simulink model "Prescan_Carsim_0118_repair_cs"  (R2019b)
settings: Solver=ode5  StartTime=0.0  StopTime=inf  FixedStep=1/1000  RelTol=1e-3
PreLoadFcn:
  | mbxruntime.callbacks.PreLoadFcn(bdroot);
PostLoadFcn:
  | mbxruntime.callbacks.PostLoadFcn(bdroot);
InitFcn:
  | mbxruntime.callbacks.InitFcn(bdroot);
  | Initialization_Func;
  | %T01_Init_2106;
StartFcn:
  | mbxruntime.callbacks.StartFcn(bdroot);
  | current_sys=gcs;
  | speedblock=Simulink.findBlocks(current_sys,'Name','speed_kmh_Gain');
  | h1=add_exec_event_listener(speedblock,'PostOutputs',@SpeedVisulization);
  | outblock=Simulink.findBlocks(current_sys,'Name','trajectorycurveoutput_Gain');
  | CurveTrajectoryListenerHandle=add_exec_event_listener(outblock,'PostOutputs',@TrajectoryCurve_CallBack);
  | lanedatablock=Simulink.findBlocks(current_sys,'Name','LaneData_Gain');
  | CurveLaneListenerHandle=add_exec_event_listener(lanedatablock,'PostOutputs',@CurveLane_CallBack);
StopFcn:
  | mbxruntime.callbacks.StopFcn(bdroot);
model workspace: external: MAT-File .\Prescan_Carsim_1230_cs_hws.mat (data not in the file)
undefined symbols (not defined in the file or in its folder): AAx, AAy, AAz, AVx, AVy, AVz, Ax, Ay, Az, canChannel, DiscIntNeverNeededParam, g, InitialDPMPDF_Comfort, InitialDPMPDF_Efficiency, InitialDPMPDF_Safety, InitialPDF_DEM, InitialPlanningParameter, Kf, Kr, Lr, M, mbxruntime, nG, NormalisedTrajectoryIndicator_Pool, Parameter_Indicator_LookUpTable, Prescan_Carsim_1230_cs_0658e9ca1334a8be, Prescan_Carsim_1230_cs_08c5eb9a1bd7376a, Prescan_Carsim_1230_cs_6cfd759b89b9fc85, Prescan_Carsim_1230_cs_9435cc1cceb5050d, Prescan_Carsim_1230_cs_ac716d34d49f74ab, Prescan_Carsim_1230_cs_be02757d7f212dd5, Rational_Coefficient_Learning, SteeringWheel, TrajectoryIndicatorRange, V, VehicleBaseLength, Vx, Vy, Vz, WheelL0, WheelL1, WheelR0, WheelR1
libraries: canmsglib x11, dsparch4 x6, canlib x3, PreScanSimulinkLibrary x3, Solver_SF x1, autolibshared x1
(part 5 of 8)

== matlab function Prescan_Carsim_0118_repair_cs/BMW_X5_SUV_1/trajectory planning/Road data extraction ==
  data: RoadLanePoly_Rotation output; RoadLaneEnd_Rotation output; u input; PathLength_Planning input; RoadLane_Plan output double size=[1000 4]; Interval_RoadSegment input; Width_Road input
function [RoadLanePoly_Rotation,RoadLaneEnd_Rotation,RoadLane_Plan]=fcn(u,PathLength_Planning,Interval_RoadSegment,Width_Road)
% calculate the road based on the ALMS sensor
% #codegen

Labels=zeros(size(u,1) , 1);
Lengths = zeros(size(u,1) , 1);
GroupIDs = zeros(size(u,1) , 1);
Pxs = zeros(size(u,1) , 4);
Pys = zeros(size(u,1) , 4);

for i = 1 : size(u,1)  
    % The valid parameter indicates that the data slot in the bus is actually filled in
    if u(i).HEADER.valid == 1         
        Labels(i)=u(i).DATA.LineLabel;
        Lengths(i) = u(i).DATA.Length; 
        GroupIDs(i) =u(i).DATA.GroupID;       
        % Count the number of groups. Polynomials with the same GroupID are
        % published sequentially in the output, which allows us to use this
        % simple piece of code.       
        % Construct polynomial definitions 
        Pxs(i,:) = [u(i).DATA.X.N3, u(i).DATA.X.N2, u(i).DATA.X.N1, u(i).DATA.X.N0];
        Pys(i,:) = [u(i).DATA.Y.N3, u(i).DATA.Y.N2, u(i).DATA.Y.N1, u(i).DATA.Y.N0];        
    end  
end

%Left Lane
ID_Left_Lane=find(Labels==5);% the left lane is labels as 5
%Right Lane
ID_Right_Lane=find(Labels==4);% the right lane is labels as 4

% Align the left and right raod lane and cut into segments with fixed
% intervals.

% To use the path planning method, we need to Align  of Left and Right Lane.
% Method 1: Cut by the Cross Dot method by Aligning the Road_Start & the
% Road_End

% Method 2:Make a Virtual Lane with a fixed Road Width 3.75m and a fixed 
% Lane Length(==PathLength_Planning)to the Base Line.
%{
% S1,Estimate the Direction of the foward Road and to determine the Base Lane
% Direction Estimation Method:the Whole Lane is on the one side of the
% vehicle longitudinal axis 
% if Flag_Left==1, the Whole Left Lane is on the left of the vehicle
Vec_Left_Lane=[LeftLane_Vis,zeros(Num_Left,1)];
Cross_LongidVehicleAxisToLeftLane=cross(Vec_LongidVehicleAxis,Vec_Left_Lane);
Flag_Left=all(Cross_LongidVehicleAxisToLeftLane(:,3)>0);

% if Flag_Right==1, the Whole Right Lane is on the right of the vehicle
Vec_Right_Lane=[RightLane_Vis,zeros(Num_Left,1)];
Cross_LongidVehicleAxisToLeftLane=cross(Vec_LongidVehicleAxis,Vec_Right_Lane);
Flag_Right=all(Cross_LongidVehicleAxisToLeftLane(:,3)<0);
% Notice that: the Lane data coordinates is the Vehicle Coordination.
%}

% Step 1,If RightLane longer than the Path_length_Planning,Choose the Right 
% one,otherwise,choose the longer one. 
% Step 2, made the Virtual Lane with a fixed Road Width 3.75m
% LeftLane_Plan=zeros(1000,2);
% RightLane_Plan=zeros(1000,2);
Length_RightLane=sum(Lengths(ID_Right_Lane));
Length_LeftLane=sum(Lengths(ID_Left_Lane));
if Length_RightLane<PathLength_Planning && Length_RightLane<Length_LeftLane
    Flag_RightBase=0;
    if Length_LeftLane>PathLength_Planning
        %LeftLane is longer than PathLength_Planning
        [LeftLane_PlanTemp,Num_LeftLane]=RoadLane_Extract_Plan(ID_Left_Lane,Pxs,Pys,Lengths,PathLength_Planning,Interval_RoadSegment);    
    else
        [LeftLane_PlanTemp,Num_LeftLane]=RoadLane_Extract_Plan(ID_Left_Lane,Pxs,Pys,Lengths,Length_LeftLane,Interval_RoadSegment);
    end
    LeftLane_Plan=LeftLane_PlanTemp(1:Num_LeftLane,:);
    [RightLane_Plan]=Made_VirtualLane(LeftLane_Plan,Flag_RightBase,Width_Road);
else
    Flag_RightBase=1;
    if Length_RightLane>PathLength_Planning
        [RightLane_PlanTemp,Num_RightLane]=RoadLane_Extract_Plan(ID_Right_Lane,Pxs,Pys,Lengths,PathLength_Planning,Interval_RoadSegment);     
    else
        [RightLane_PlanTemp,Num_RightLane]=RoadLane_Extract_Plan(ID_Right_Lane,Pxs,Pys,Lengths,Length_RightLane,Interval_RoadSegment);
    end
    RightLane_Plan=RightLane_PlanTemp(1:Num_RightLane,:);
    [LeftLane_Plan]=Made_VirtualLane(RightLane_Plan,Flag_RightBase,Width_Road);
end

RoadLane_Plan=[LeftLane_Plan,RightLane_Plan];

% Fit the RoadLane 
Order_polyfit=6;
rotationangle=deg2rad(45);
rotationmatrix=[cos(rotationangle),sin(rotationangle);-sin(rotationangle),cos(rotationangle)];
leftlane_rotation=LeftLane_Plan*rotationmatrix;
Poly_LeftRotation=polyfit(leftlane_rotation(:,1),leftlane_rotation(:,2),Order_polyfit);
rightlane_rotation=RightLane_Plan*rotationmatrix;
Poly_RightRotation=polyfit(rightlane_rotation(:,1),rightlane_rotation(:,2),Order_polyfit);
RoadLanePoly_Rotation=[Poly_LeftRotation',Poly_RightRotation'];
RoadLaneEnd_Rotation=[leftlane_rotation(end,:),rightlane_rotation(end,:)];

end

%%
% Local functions
function [Temp_Lane,Num_Lane]=RoadLane_Extract_Vis(ID_Lane,Num_short_length,Pxs,Pys,Lengths)
% Extract Lane data according to the Polyvals from ALMS
% Input: 
%   Num_short_length, when the road length of a poly short than this 
%       this value, the polyval is evaluated with a smaller interval
%   Pxs,Pys, the poly coefficients for X,Y
Temp_Lane=zeros(5000,2);% a large vector used to store the data
Num_Lane=0;
for i=1:length(ID_Lane)
    road_length=Lengths(ID_Lane(i)); 
    if road_length<1
        L = linspace(0,road_length,Num_short_length);
    else
        L = 0:0.1:road_length;
    end        
    X_temp = polyval(Pxs(ID_Lane(i),:),L);
    Y_temp = polyval(Pys(ID_Lane(i),:),L);        
    Num_point=length(L);        
    Temp_Lane(Num_Lane+1:Num_Lane+Num_point,1)=X_temp';
    Temp_Lane(Num_Lane+1:Num_Lane+Num_point,2)=Y_temp';
    Num_Lane=Num_Lane+Num_point;
end
end

function [Lane_Plan,Num_RoadSegment]=RoadLane_Extract_Plan(ID_Lane,Pxs,Pys,Lengths,LaneLength,Interval_RoadSegment)
% Extract Lane data according to the Polyvals from ALMS
% Input: 
%   Pxs,Pys, the poly coefficients for X,Y
%   PathLength, the target path length 
%   Interval_RoadSegmetn,choose the raod point with a length interval.
Lane_Plan=zeros(1000,2);
LengthPoint=0:Interval_RoadSegment:LaneLength;
Num_RoadSegment=length(LengthPoint);
CumSum_LengthLane=cumsum([0;Lengths(ID_Lane)]);
% the First Road segment point
Lane_Plan(1,1)= polyval(Pxs(ID_Lane(1),:),0);
Lane_Plan(1,2)= polyval(Pys(ID_Lane(1),:),0); 
for i=2:Num_RoadSegment
    LengthPoint_i=LengthPoint(i);
    ID_Close=find(LengthPoint_i<=CumSum_LengthLane);
    ID_poly=ID_Close(1,1)-1;        
    Lane_Plan(i,1) = polyval(Pxs(ID_Lane(ID_poly),:),LengthPoint_i-CumSum_LengthLane(ID_poly));
    Lane_Plan(i,2) = polyval(Pys(ID_Lane(ID_poly),:),LengthPoint_i-CumSum_LengthLane(ID_poly));                       
end
end

function [Lane_Virtual]=Made_VirtualLane(BaseLane,Flag_RightBase,Width_Road)
% made the virtual lane based on the baselane with a fixed road width
% 3.75m.
% BaseLane: a array like Num_roadpoint*2,the first column is the X
% coordinates while the other column is the Y coordinates.
% Flag_Right:a logical variable, if 1, it shows the baselane is the right
% one, if 0, the baselane is the left one.
% Lane_Virtual=zeros(1000,2);% a large data array to fix the size of the output.
Vec_BaseLane=zeros(size(BaseLane,1),2);
Vec_BaseLane(1:end-1,1)=BaseLane(2:end,1)-BaseLane(1:end-1,1);
Vec_BaseLane(end,1)=Vec_BaseLane(end-1,1);
Vec_BaseLane(1:end-1,2)=BaseLane(2:end,2)-BaseLane(1:end-1,2);
Vec_BaseLane(end,2)=Vec_BaseLane(end-1,2);
VecLength_BaseLane=sqrt(Vec_BaseLane(:,1).^2+Vec_BaseLane(:,2).^2);
Vec_BaseLane_unit=[Vec_BaseLane(:,1)./VecLength_BaseLane,Vec_BaseLane(:,2)./VecLength_BaseLane];
if Flag_RightBase==1
    Rotation_Transformation=[0,-1;1,0];
else
    Rotation_Transformation=[0,1;-1,0];
end
Vec_VirtualToBase=Rotation_Transformation*Vec_BaseLane_unit';% 2*N
Lane_Virtual=BaseLane+Width_Road*Vec_VirtualToBase';

end



%{
function [Flag_Cut,SecondLane_AfterCut]=Road_Align(FirstLane,SecondLane,Rotation_Angle_deg)
% Function:Align the Road_Start & the Road_End
% Method: Cut by the Cross Dot method
% Input: Rotation_Angle=90 for the FirstLane is the Right lane;
%        Rotation_Angle=-90 for the FirstLane is the Left lane.
%        FisrtLane or SecondLane is a data array like Num*2, the first column is the X
%        coordinates,and the second column is the Y coordinates.
Num_Second=size(SecondLane,1);

Vec_First_Start=zeros(1,3);
Vec_First_Start(1,1:2)=FirstLane(2,:)-FirstLane(1,:);
% clock-wise (Negative) for Left Lane to rotate
% Rotation_Angle=deg2rad(-90);
% Rotation_Angle=deg2rad(Rotation_Angle_deg);
Rotation_Transformation=[cos(Rotation_Angle),-1*sin(Rotation_Angle);sin(Rotation_Angle),cos(Rotation_Angle)];

Vec_SecondToFirstStart=zeros(Num_Second,3);
Vec_SecondToFirstStart(:,1:2)=SecondLane-FirstLane(1,:);

Vec_VerticalToFirstStart=[Rotation_Transformation*Vec_First_Start(1,1:2)';0];
Vec_VerticalToFirstStart_Matrix=repmat(Vec_VerticalToFirstStart',Num_Second,1);
Cross_VerticalToLeftStart=cross(Vec_VerticalToFirstStart_Matrix,Vec_SecondToFirstStart);
% Find the road point that lies out of the Vec_VerticalToLeftStart
ID_FirstStart=find(Cross_VerticalToLeftStart(:,3)*sign(Rotation_Angle)>0);
if isempty(ID_FirstStart)
    Flag_Cut=0;    
    SecondLane_AfterCut=SecondLane;
else
    Flag_Cut=1;
    SecondLane_AfterCut=SecondLane(ID_FirstStart(end)+1:end,:);   
end
end
%}

== matlab function Prescan_Carsim_0118_repair_cs/BMW_X5_SUV_1/Tracking Control & vehicle dynamics/Lane Keeping Assistance/Path Tracking - LQR controller/LQR Feedforward ==
  data: Feedforward output; PreviewDistance input; Curvature input; v input
function Feedforward = fcn(PreviewDistance, Curvature,v)
% LQR前馈量计算，与赵斌的SMC前馈量计算完全一致
%先定义车辆本身的参数
g=9.8;%重力加速度m/s^2

%=============== Original Vehicle Parameters
M=1396; %车辆的质量kg
I=2204; %车辆的横摆转动惯量kg·m2
Kf=50192; %前轮的侧偏刚度Nm/rad
Kr=50192; %后轮的侧偏刚度Nm/rad
Lf=1.01; %车辆质心到前轴的距离m
Lr=1.59; %车辆质心到后轴的距离m
%{
%=====The JTEKT vehicle Parameter
M=1275; %车辆的质量kg
I=1523; %车辆的横摆转动惯量kg·m2
Kf=20000; %Calculated According to the carsim vehicle tire (under Fn=3500N)
Kr=20000; %后轮的侧偏刚度Nm/rad
Lf=1.016; %车辆质心到前轴的距离m
Lr=1.644; %车辆质心到后轴的距离m
%}


%待调参数： 预瞄时长t_pre, 滑膜面参数 c1, c2, 趋近率参数delta, kapa
%输入参数； 预瞄偏差ep,  参考航向角phi_d, 本车航向角 phi, 道路曲率 qulv  航向角偏差影响系数 phir_k0 phir_k1
L = PreviewDistance; %车辆预瞄距离设定
smc_a34 = (Kf+Kr)/M+L*(Kf*Lf-Kr*Lr)/I;
smc_b32 = (L*Kf*Lf)/I+Kf/M;
k3 = smc_a34/smc_b32;
Feedforward= (M*v^2*Curvature)/(2*(Lf+Lr))*(Lr/Kf-Lf/Kr+Lf/Kr*k3)+Curvature*((Lf+Lr)-Lr*k3);

== matlab function Prescan_Carsim_0118_repair_cs/BMW_X5_SUV_1/trajectory planning/Specific Curve Trajectory Planning/Trajectory Planning For Curve under beginning-global/Trajectory Planning For Curve ==
  data: RoadLane_Plan input size=[1000 4]; PathPlan_Global output size=[1000 2]; Parameter_TrajectoryPlan input size=[9 1]; Speed_Planned_kmh output size=[1000 1]; VehicleWidth input; LaneWidth input; PlanPathDataLength_Curve output size=1; VehicleState_Beginning input
function [PathPlan_Global,Speed_Planned_kmh,PlanPathDataLength_Curve]= fcn(RoadLane_Plan,Parameter_TrajectoryPlan,VehicleWidth,LaneWidth,VehicleState_Beginning)
%Road Lane
Path_PlanTemp=zeros(1000,2);
Num_LanePlan=size(RoadLane_Plan,1);
LeftLane_Plan=RoadLane_Plan(:,1:2);
RightLane_Plan=RoadLane_Plan(:,3:4);
X_LaneLeftToRight=RightLane_Plan(:,1)-LeftLane_Plan(:,1);
Y_LaneLeftToRight=RightLane_Plan(:,2)-LeftLane_Plan(:,2);
Vec_LeftToRight=[X_LaneLeftToRight,Y_LaneLeftToRight];
LaneWidth_Estimated=sqrt(sum(Vec_LeftToRight.*Vec_LeftToRight,2));
UnitVec_LeftRight=Vec_LeftToRight./[LaneWidth_Estimated,LaneWidth_Estimated];
LaneCenter=zeros(Num_LanePlan,2);
LaneCenter(:,1)=0.5*(LeftLane_Plan(:,1)+RightLane_Plan(:,1));
LaneCenter(:,2)=0.5*(LeftLane_Plan(:,2)+RightLane_Plan(:,2));
LeftBound=LaneCenter-(LaneWidth-VehicleWidth)*0.5*UnitVec_LeftRight; % The Path Bound Should consider the Vehicle Width
RightBound=LaneCenter+(LaneWidth-VehicleWidth)*0.5*UnitVec_LeftRight;

%path planning
% Trajectory planning parameters
Init_pos=0.5;
Parameter_PathPlan=Parameter_TrajectoryPlan(1:4,1);
if sum(Parameter_TrajectoryPlan(1:3)>1)
    Parameter_PathPlan=[0,0,1,0.5];
end
% if Parameter_PathPlan(3)==1
%     alpha=ones(Num_LanePlan,1)*Parameter_PathPlan(4);
%     alpha(1:2)=Init_pos;
%     alpha(end-1:end)=Init_pos;  
% else
[alpha_path_length,alpha_curvature,~,~,G]= PathPlanning(RightBound(:,1),...
    RightBound(:,2),LeftBound(:,1),LeftBound(:,2),Init_pos);
% fixed lateral offst
alpha_fixlatoff=ones(Num_LanePlan,1)*Parameter_PathPlan(4);
sign_center=sign(Parameter_PathPlan(4)-Init_pos);
offset=0.02;
alpha_fixlatoff(1:3)=Init_pos;% consistent within the pathplanning function
alpha_fixlatoff(4:21)=pchip([1,5,14,18],[Init_pos,Init_pos+sign_center*offset,Parameter_PathPlan(4)-sign_center*offset,Parameter_PathPlan(4)],(1:18));
alpha_fixlatoff(end-2:end)=Init_pos;
% alpha_heading(4:6)=spline([1,5],[Init_pos,Parameter_PathPlan(4)],(2:4));
% alpha_heading(end-5:end-3)=spline([1,5],[Parameter_PathPlan(4),Init_pos],(2:4));
alpha_fixlatoff(end-20:end-3)=pchip([1,5,14,18],[Parameter_PathPlan(4),Parameter_PathPlan(4)-sign_center*offset,Init_pos+sign_center*offset,Init_pos],(1:18));

alpha=[alpha_path_length,alpha_curvature,alpha_fixlatoff]*Parameter_PathPlan(1:3,1);% Num_roadseg*Num_beta
% end
Path_PlanTemp(1:Num_LanePlan,1) = RightBound(:,1) + (LeftBound(:,1)-RightBound(:,1)).* alpha;
Path_PlanTemp(1:Num_LanePlan,2)= RightBound(:,2) + (LeftBound(:,2)-RightBound(:,2)).* alpha;
Path_Plan_Local=Path_PlanTemp;
PlanPathDataLength_Curve=Num_LanePlan;

% Convert the Local path to global path
PathPlan_Global=Transfer2Global(Path_Plan_Local,VehicleState_Beginning);
% HeadingAngle_Beginning_rad=VehicleState_Beginning(3);
% Rotation_Beginning=[cos(HeadingAngle_Beginning_rad),-sin(HeadingAngle_Beginning_rad); sin(HeadingAngle_Beginning_rad),cos(HeadingAngle_Beginning_rad)];
% PathPlan_Beginning_temp=Path_Plan_Local(:,1:2)*Rotation_Beginning';
% PathPlan_Global=[PathPlan_Beginning_temp(:,1)+VehicleState_Beginning(1),...
%     PathPlan_Beginning_temp(:,2)+VehicleState_Beginning(2)];

% Speed_Profile planning
% step 1, Calculate the curvature of the path
Curvature=Curvature_cal(Path_Plan_Local(1:Num_LanePlan,1),Path_Plan_Local(1:Num_LanePlan,2));
Curvature(1:10)=0;
Curvature(end-9:end)=0;

Parameter_SpeedPlan=Parameter_TrajectoryPlan(5:end,1);
% The speed plan parameters
LatAcceleration_Limit=Parameter_SpeedPlan(1);% m/s2
LongidAcceleration_Limit=Parameter_SpeedPlan(2);% m/s2
LongidDeceleration_Limit=Parameter_SpeedPlan(3);% m/s2
Velocity_LowerBound=Parameter_SpeedPlan(4)/3.6;% m/s
Velocity_UpperBound=Parameter_SpeedPlan(5)/3.6;% m/s
% Begin speed plan
Speed_Planned_kmh=zeros(1000,1);

SpeedProfile_Temp=Speedprofile(Num_LanePlan,Curvature,LatAcceleration_Limit,LongidAcceleration_Limit,...
LongidDeceleration_Limit,Velocity_LowerBound,Velocity_UpperBound,G);% the speedProfile is a 1000*1 data array
% smooth the speed
% span = 5;
% SpeedProfile_Temp=smooth_solver(SpeedProfile_Temp,span);
Speed_Planned_kmh(1:Num_LanePlan,1)=SpeedProfile_Temp*3.6;% km/h

end


%%
% Local functions
function [alpha_path_length,alpha_curvature,alpha_centering,alpha_heading_error,G]= PathPlanning(Xr,Yr,Xl,Yl,Init_pos)
% alpha_path_length: the solution of the shortest path
% alpha_curvature:the solution of the minimum curvature
% alpha_centering:the solution of the centering 
% alpha_heading_error:the solution of the minimum heading error
Num_point=size(Xr,1);

% lb = zeros(size(Xr,1),1);
lb = 0.2*ones(size(Xr,1),1);
ub = 0.80*ones(size(Xr,1),1);
lb(1:3) = Init_pos;
ub(1:3)=Init_pos;
lb(end-2:end) = Init_pos;
ub(end-2:end)=Init_pos;
%     lb(end) = 0.5;
%     ub(end) = 0.5;

delta_X = Xl - Xr;% (n+1)*1
delta_Y = Yl - Yr;
% Quadratic programming
% objective function of minimum distance
H_dist = diag(2*delta_X.*delta_X)+diag(-delta_X(1:end-1).*delta_X(2:end),-1)...
    +diag(-delta_X(1:end-1).*delta_X(2:end),1)+diag(2*delta_Y.*delta_Y)...
    +diag(-delta_Y(1:end-1).*delta_Y(2:end),-1)...
    +diag(-delta_Y(1:end-1).*delta_Y(2:end),1);
H_dist(1, 1) = delta_X(1).*delta_X(1)+delta_Y(1).*delta_Y(1);
H_dist(end, end) = delta_X(end).*delta_X(end)+delta_Y(end).*delta_Y(end);
B_dist_con = diag(ones(1,Num_point)*4)...
    +diag(ones(1,Num_point-1)*-2,-1)+diag(ones(1,Num_point-1)*-2,1);
B_dist_con(1,1) = 2; B_dist_con(end,end) = 2;
B_dist = diag(delta_X)*B_dist_con*Xr + diag(delta_Y)*B_dist_con*Yr;
H_dist_qp = H_dist * 2;
alpha_path_length = activeset_bc_simple(H_dist_qp,B_dist,lb,ub);

% objective function of minimum curvature
M = diag(ones(1,Num_point)*4)+diag(ones(1,Num_point-1),-1)+diag(ones(1,Num_point-1),1);
M(1,1) = 2; 
M(end,end) = 2;
N = diag(ones(1,Num_point-1)*-1,-1)+diag(ones(1,Num_point-1),1);
N(1,1) = -1; N(end,end) = 1;
O = diag(ones(1,Num_point)*-1)+diag(ones(1,Num_point-1),1);
O(end,:) = [];
P=diag(ones(1,Num_point)*2)+diag(ones(1,Num_point-1),1);
P(end,:) = [];
D = 6 * (O - P* pinv(M) * N);
G = 3 * pinv(M)*N;
H_tao=diag(delta_X)'*(D'*D)*diag(delta_X) + diag(delta_Y)'*(D'*D)*diag(delta_Y);
B_tao=(2*Xr'*(D'*D)*diag(delta_X) + 2*Yr'*(D'*D)*diag(delta_Y))';
H_tao_qp = H_tao*2;
alpha_curvature = activeset_bc_simple(H_tao_qp,B_tao,lb,ub);

% objective function of minimum heading error
H_P = diag(2*ones(1,Num_point))+diag(-1*ones(1,Num_point-1),1)+diag(-1*ones(1,Num_point-1),-1);%(n+1)*(n+1)
H_P(1,1)=1;
H_P(end,end)=1;
B_HeadingError = zeros(size(Xr,1),1);
H = 2*H_P;
alpha_heading_error = activeset_bc_simple(H,B_HeadingError,lb,ub);

alpha_centering=0.5*ones(size(Xr,1),1);
alpha_centering(1) = Init_pos;
%alpha_centering(2:end) = 0.5;
%alpha = beta_path_length*alpha1 + beta_curvature*alpha2 + beta_centering*alpha3 + (1-beta_path_length-beta_curvature-beta_centering)*alpha4;
end

function yy = smooth_solver(y,span)
    %method: Moving Average 
    %Maintain by HoGinhang
%     n = size(y,1);
    n = length(y);
    hw=floor(span/2);
    yy=y;
    for i = 2:n
        if(i<=hw)
            k1 = 1;
            k2 = 2*(i-k1)+1;
            z = k2;
        elseif((i+hw)>=n)
            k1 = 2*i-n;
            k2 = n;
            z = k2-k1+1;
        else
            k1 = i-hw;
            k2 = i+hw;
            z = span;
        end
        tmp=sum(y(k1:k2));
        yy(i) = tmp/z;
    end
    yy=yy';
end

function Lane_Global=Transfer2Global(Lane_Local,GlobalState_LocalOrigin)
% GlobalState_LocalOrigin:is a tripple element array(X,Y,Yaw),Yaw_rad
HeadingAngle_Beginning_rad=GlobalState_LocalOrigin(3);
Rotation_Beginning=[cos(HeadingAngle_Beginning_rad),-sin(HeadingAngle_Beginning_rad); sin(HeadingAngle_Beginning_rad),cos(HeadingAngle_Beginning_rad)];
PathPlan_Beginning_temp=Lane_Local(:,1:2)*Rotation_Beginning';
Lane_Global=[PathPlan_Beginning_temp(:,1)+GlobalState_LocalOrigin(1),...
    PathPlan_Beginning_temp(:,2)+GlobalState_LocalOrigin(2)];


end

function cur_fro = Curvature_cal(XtsTem,YtsTem)
Num_path=size(XtsTem,2);
cur_fro = zeros(size(XtsTem));
span_smooth = 6;% used to smooth the curvature
for j=1:Num_path
    for i = 1:size(XtsTem,1)
        if (i == 1)
            x = [XtsTem(i,j);XtsTem(i+1,j);XtsTem(i+2,j);XtsTem(i+3,j);XtsTem(i+4,j)];
            speed = [YtsTem(i,j);YtsTem(i+1,j);YtsTem(i+2,j);YtsTem(i+3,j);YtsTem(i+4,j)];
        elseif (i == 2)
            x = [XtsTem(i-1,j);XtsTem(i,j);XtsTem(i+1,j);XtsTem(i+2,j);XtsTem(i+3,j)];
            speed = [YtsTem(i-1,j);YtsTem(i,j);YtsTem(i+1,j);YtsTem(i+2,j);YtsTem(i+3,j)];
        elseif (i == size(XtsTem,1)-1)
            x = [XtsTem(i-3,j);XtsTem(i-2,j);XtsTem(i-1,j);XtsTem(i,j);XtsTem(i+1,j)];
            speed = [YtsTem(i-3,j);YtsTem(i-2,j);YtsTem(i-1,j);YtsTem(i,j);YtsTem(i+1,j)];
        elseif (i == size(XtsTem,1))
            x = [XtsTem(i-4,j);XtsTem(i-3,j);XtsTem(i-2,j);XtsTem(i-1,j);XtsTem(i,j)];
            speed = [YtsTem(i-4,j);YtsTem(i-3,j);YtsTem(i-2,j);YtsTem(i-1,j);YtsTem(i,j)];
        else
            x = [XtsTem(i-2,j);XtsTem(i-1,j);XtsTem(i,j);XtsTem(i+1,j);XtsTem(i+2,j)];
            speed = [YtsTem(i-2,j);YtsTem(i-1,j);YtsTem(i,j);YtsTem(i+1,j);YtsTem(i+2,j)];
        end
%             cur_fro(i,j) = rwqulv(x,y); 
        A=[x,speed,ones(length(x),1)];
        if rank(A) ~= size(A,2)
            cur_fro(i,j) = 0;
        else
            B=-1*(x.^2+speed.^2);
            coef=A\B;%圆一般方程式的的系数DEF
            cur_fro(i,j)= 2/sqrt(coef(1)^2+coef(2)^2-4*coef(3));
        end
    end  
    cur_fro(:,j)= smooth_solver(cur_fro(:,j),span_smooth);
end
end


function Speed_PlannedTemp=Speedprofile(Num_point,Curvature,a_latlim,a_acclim,a_declim,v_min_con,v_max_con,G)

coder.extrinsic('quadprog','optimoptions');  
% lb_1 = [];
% ub_1 = [];
miu=0.8;% the Road adhesion coefficient
g=9.8;% m/s2,the Gravity coefficient

v_max_TierAdLimit=sqrt(miu * g ./ (Curvature+eps));%upper bounds by tier adhesion limit
ub_Curvature = sqrt(1 ./ (abs(Curvature)+eps) .* a_latlim);% upper bounds by Parameter_LatAcceleration
ub_Parameter = v_max_con .* ones(Num_point,1);%speed upper bound from Parameter_SpeedPlan
lb_Parameter = v_min_con .* ones(Num_point,1);%speed lower bound from Parameter_SpeedPlan

UpperBound =min([ub_Curvature,ub_Parameter],[],2);
UpperBound=max([UpperBound,lb_Parameter],[],2)+0.1;
LowerBound = lb_Parameter;

v_MaxTarget = min(v_max_TierAdLimit,ub_Parameter);
H_QuadObjective = 2 * eye(Num_point);% quadratic obejective term
f_LinearObjective = -2 * v_MaxTarget';% Linear obejective term
A_InequallityConstraint = [G.*2;-G.*2];% Linear inequallity constraints
b_InequallityConstraint= [a_acclim .* ones(Num_point,1);a_declim .* ones(Num_point,1)];% Linear Inequality constraints
% Speed_Planned=zeros(1000,1);
options = optimoptions('quadprog','Display','off');
Speed_PlannedTemp = quadprog(H_QuadObjective,f_LinearObjective,A_InequallityConstraint,b_InequallityConstraint,[],[],LowerBound,UpperBound,[],options);% There is no equality constraints 
% Speed_Planned(1:Num_point,1)=Speed_PlannedTemp;

end

function x=activeset_bc_simple(H,g,LB,UB)
%
% Active set algorithm for quadratic program with bound constraints. 
% [x,lam,ws,oc,cc]=activeset_bc(H,g,LB,UB,tol,maxiter), solves the 
% strictly convex quadratic program of the form
%
% min 0.5x'*H*x+g'*x, s.t. LB<=x<=UB, 
%
% where H=H'>0. 
%
% [x,lam,ws,oc,cc]=activeset_bc(H,g,LB,UB), work with default parameters.
% 
% This is modification of the algorithm 16.3 from Nocedal & Wright , p. 472.
% Input:
% H - positive definite and symmetric hessian matrix (nxn).
% g - vetor (nx1).
% tol - tolerance for equality constrained subproblem (16.39), p. 468 in N&W, (Default: 10^(-12)) 
% maxiter - max. number of main iterations, (Default: 100*length(x))
% Output: 
% x  - optimal solution.
% f=0.5x'*H*x+g'*x - minimum function value 
% lam(k) - Lagrange multiplier corresponding to LB(k)<=x(k)<=UB(k), k=1,..,n.
% ws - is an optimal active set. If ws(k)=-1, then x(k)=LB(k). If ws(k)=+1,
% then x(k)=UB(k), otherwise ws(k)=0.
% oc - is an optimality measure i.e. ||Lx||=||H*x+g-A'*lam||, where
% the Lagrangian
%
% L=0.5x'*H*x+g'*x-lam'*(A*x-b),
%
% and A=[I;-I], b=[LB;-UB].
%
% cc - is complementarity measure i.e.
%
% cc = max  |lam(i)*min(x(i)-LB(i),UB(i)-x(i))|
%    i=1,..,n
%
% The activeset_bc, is usually (but not always), faster than quadprog/interior-point 
% To compare with quadprog/interior-point try to run the following code:

% (C) 2021, by dr Piotr Bania, pba@agh.edu.pl.
% http://home.agh.edu.pl/~pba/

n=length(g);
LB=LB(:);UB=UB(:);g=g(:);
[nh,mh]=size(H);nlb=length(LB);nub=length(UB);
s=(nh==mh && n==nh && n==nub && n==nlb);
if ~s
    x=0.5*ones(n,1);
    return
end
tol=1e-10;
maxiter=100*n;

k=0;stop=0;
opts.SYM =true;opts.POSDEF=true;opts.TRANSA=false;
x=linsolve(H,-g,opts); % Compute global solution.
x=max(LB,x);x=min(UB,x); % Starting point.
% Working set. 
% If x(k)=LB(k)-->ws(k)=-1, elseif x(k)=UB(k)-->ws(k)=+1,else --> ws(k)=0. 
ws=zeros(n,1);ws(x==LB)=-1;ws(x==UB)=1;
% If ws is empty -->stop, global solution LB<x=-H^(-1)g<UB.
if max(abs(ws))==0
    stop=1;
end
while ~stop
    gk=H*x+g; % Compute gradient.
    ind=find(ws==0); % Identify free variables.
    if isempty(ind) % If all constraints are active.
        % Trivial solution of the equality constrained subproblem. 
        pk=zeros(n,1);
        lam=-ws.*gk; % Compute Lagrange multipliers.
    else
        % Solution of the equality constrained subproblem.
        Hr=H(ind,ind);gr=gk(ind); % Reduced hessian and gradient. 
        pr=linsolve(Hr,-gr,opts); % Solution of the reduced subproblem. 
        pk=zeros(n,1);pk(ind)=pr; % Solution of the subproblem. 
        lam=-ws.*(H*pk+gk); % Compute Lagrange multipliers, A'*lam=H*pk+gk.
    end
    if norm(pk)<tol % If pk==0, i.e. the subproblem has trivial solution.
        if min(lam)>=0  
            stop=1; % If all multipliers are non-negative --> stop.
        else
            ws(lam<0)=0; % Remove constraints with negative multipliers.
        end
    else
        % Max step and blocking constraint
        [al,jblock,sg]=get_max_step(x,pk,LB,UB,n);
        if jblock>0 % If there are some blocking constraint.
            ws(jblock)=sg; % Add blocking constraint to ws.
        end
        x=x+al*pk; % Step
    end
    k=k+1;
    if k>maxiter % If max. number of iteration
        stop=1;
    end
end
end

function [al,j,s]=get_max_step(x,pk,LB,UB,n)
% Compute max. step s.t LB<=x+al*pk<=UB && 0<=al<=1.
% j - index of blocking constraint,
% s=1, upper bound is active , s=-1 - lower bound is active
% If LB<x+pk<UB, then al=1, j=0, s=0 - no blocking constraits
al=1;j=0;s=0;
for i=1:n
    if pk(i)>0
        altmp=(UB(i)-x(i))/pk(i);stmp=1;
    elseif pk(i)<0
        altmp=(LB(i)-x(i))/pk(i);stmp=-1;
    else
        altmp=inf;stmp=0;
    end
    if altmp<al
        al=altmp;j=i;s=stmp;  
    end
end
end

== matlab function Prescan_Carsim_0118_repair_cs/BMW_X5_SUV_1/trajectory planning/A substitution for the above trajectory planning subsystem/Trajectory Planning For Curve under beginning-global/Trajectory Planning For Curve ==
  data: RoadLane_Plan input size=[1000 4]; Path_Plan output size=[1000 2]; Parameter_TrajectoryPlan input size=[9 1]; Speed_Planned_kmh output size=[1000 1]; VehicleWidth input; LaneWidth input; PlanPathDataLength_Curve output size=1
function [Path_Plan,Speed_Planned_kmh,PlanPathDataLength_Curve]= fcn(RoadLane_Plan,Parameter_TrajectoryPlan,VehicleWidth,LaneWidth)
coder.extrinsic('smooth');

%Road Lane
Path_PlanTemp=zeros(1000,2);
Num_LanePlan=size(RoadLane_Plan,1);
LeftLane_Plan=RoadLane_Plan(:,1:2);
RightLane_Plan=RoadLane_Plan(:,3:4);
X_LaneLeftToRight=RightLane_Plan(:,1)-LeftLane_Plan(:,1);
Y_LaneLeftToRight=RightLane_Plan(:,2)-LeftLane_Plan(:,2);
Vec_LeftToRight=[X_LaneLeftToRight,Y_LaneLeftToRight];
LaneWidth_Estimated=sqrt(sum(Vec_LeftToRight.*Vec_LeftToRight,2));
UnitVec_LeftRight=Vec_LeftToRight./[LaneWidth_Estimated,LaneWidth_Estimated];
LaneCenter=zeros(Num_LanePlan,2);
LaneCenter(:,1)=0.5*(LeftLane_Plan(:,1)+RightLane_Plan(:,1));
LaneCenter(:,2)=0.5*(LeftLane_Plan(:,2)+RightLane_Plan(:,2));
LeftBound=LaneCenter-(LaneWidth-VehicleWidth)*0.5*UnitVec_LeftRight; % The Path Bound Should consider the Vehicle Width
RightBound=LaneCenter+(LaneWidth-VehicleWidth)*0.5*UnitVec_LeftRight;

%path planning
% Trajectory planning parameters
Init_pos=0.5;
Parameter_PathPlan=Parameter_TrajectoryPlan(1:4,1);
[alpha_path_length,alpha_curvature,alpha_centering,alpha_heading_error,G]= PathPlanning(RightBound(:,1),...
    RightBound(:,2),LeftBound(:,1),LeftBound(:,2),Init_pos);
alpha=[alpha_path_length,alpha_curvature,alpha_centering,alpha_heading_error]*Parameter_PathPlan;% Num_roadseg*Num_beta
Path_PlanTemp(1:Num_LanePlan,1) = RightBound(:,1) + (LeftBound(:,1)-RightBound(:,1)).* alpha;
Path_PlanTemp(1:Num_LanePlan,2)= RightBound(:,2) + (LeftBound(:,2)-RightBound(:,2)).* alpha;
Path_Plan=Path_PlanTemp;
PlanPathDataLength_Curve=Num_LanePlan;

% Speed_Profile planning
% step 1, Calculate the curvature of the path
Curvature=Curvature_cal(Path_Plan(1:Num_LanePlan,1),Path_Plan(1:Num_LanePlan,2));
Parameter_SpeedPlan=Parameter_TrajectoryPlan(5:end,1);
% The speed plan parameters
LatAcceleration_Limit=Parameter_SpeedPlan(1);% m/s2
LongidAcceleration_Limit=Parameter_SpeedPlan(2);% m/s2
LongidDeceleration_Limit=Parameter_SpeedPlan(3);% m/s2
Velocity_LowerBound=Parameter_SpeedPlan(4)/3.6;% m/s
Velocity_UpperBound=Parameter_SpeedPlan(5)/3.6;% m/s
% Begin speed plan
Speed_Planned_kmh=zeros(1000,1);
SpeedProfile_Temp=Speedprofile(Num_LanePlan,Curvature,LatAcceleration_Limit,LongidAcceleration_Limit,...
LongidDeceleration_Limit,Velocity_LowerBound,Velocity_UpperBound,G);% the speedProfile is a 1000*1 data array
Speed_Planned_kmh(1:Num_LanePlan,1)=SpeedProfile_Temp*3.6;% km/h
% smooth the speed
span = 4;
Speed_Planned_kmh=smooth(Speed_Planned_kmh,span);

% Construct the trajectory
% Speed_Planned=zeros(Num_LanePlan,1);
%Trajectory=[Path_Plan,Speed_Planned_kmh];

% smooth or interplate the trajecotry 

end


%%
% Local functions
function [alpha_path_length,alpha_curvature,alpha_centering,alpha_heading_error,G]= PathPlanning(Xr,Yr,Xl,Yl,Init_pos)
% alpha_path_length: the solution of the shortest path
% alpha_curvature:the solution of the minimum curvature
% alpha_centering:the solution of the centering 
% alpha_heading_error:the solution of the minimum heading error
coder.extrinsic('quadprog','optimoptions');
Num_point=size(Xr,1);
alpha_path_length=zeros(Num_point,1);
alpha_curvature=zeros(Num_point,1);
% alpha_centering=zeros(Num_point,1);
alpha_heading_error=zeros(Num_point,1);

M = zeros(Num_point,Num_point);
for i =1:Num_point
    if i == 1
        M(i,1) = 2;
        M(i,2) = 1;
    elseif i == Num_point
        M(i,Num_point-1) = 1;
        M(i,Num_point) = 2;
    else
        M(i,i-1) = 1;
        M(i,i) = 4;
        M(i,i+1) = 1;
    end
end

N = zeros(Num_point,Num_point);
for i =1:Num_point
    if i == 1
        N(i,1) = -1;
        N(i,2) = 1;
    elseif i == Num_point
        N(i,Num_point-1) = -1;
        N(i,Num_point) = 1;
    else
        N(i,i-1) = -1;
        N(i,i) = 0;
        N(i,i+1) = 1;
    end
end

O = zeros(Num_point-1,Num_point);
for i = 1:Num_point-1
    O(i,i) = -1;
    O(i,i+1) = 1;
end

P = zeros(Num_point-1,Num_point);
for i = 1:Num_point-1
    P(i,i) = 2;
    P(i,i+1) = 1;
end

D = 6 * (O - P* inv(M) * N);
G = 3 * inv(M)*N;

% objective function of minimum distance
delta_X = Xl - Xr;% (n+1)*1
delta_Y = Yl - Yr;

delta_X_ba = zeros(size(delta_X,1)-1,2);% n*2
for i = 1:size(delta_X,1)-1
    delta_X_ba(i,1) = delta_X(i+1);
    delta_X_ba(i,2) = -delta_X(i);
end

delta_Y_ba = zeros(size(delta_Y,1)-1,2);% n*2
for i = 1:size(delta_Y,1)-1
    delta_Y_ba(i,1) = delta_Y(i+1);
    delta_Y_ba(i,2) = -delta_Y(i);
end

delta_X_r = zeros(size(delta_X,1)-1,1);% n*1
for i = 1:size(delta_X,1)-1
    delta_X_r(i,1) = Xr(i+1,1) - Xr(i,1);
end

delta_Y_r = zeros(size(delta_Y,1)-1,1);% n*1
for i = 1:size(delta_Y,1)-1
    delta_Y_r(i,1) = Yr(i+1,1) - Yr(i,1);
end

E = zeros(2*(size(Xr,1)-1),size(Xr,1));% 2n*(n+1)
for i = 1:2:2*(size(Xr,1)-1)
    E(i,(i+1)/2+1) = 1;
    E(i+1,(i+1)/2) = 1;
end

dx = zeros(size(Xr,1),size(Xr,1));% (n+1)*(n+1)
for i = 1:size(Xr,1)
    dx(i,i) = delta_X(i,1);
end

dy = zeros(size(Yr,1),size(Yr,1));% (n+1)*(n+1)
for i = 1:size(Yr,1)
    dy(i,i) = delta_Y(i,1);
end

H_S = zeros(size(Xr,1),size(Xr,1));% (n+1)*(n+1)
for i =1:size(Xr,1)-1
    H_S = H_S + E(2*i-1:2*i,:)' * (delta_X_ba(i,:)'*delta_X_ba(i,:) + delta_Y_ba(i,:)'*delta_Y_ba(i,:)) *  E(2*i-1:2*i,:);
end

B_S = zeros(1,size(Xr,1));% (n+1)*(n+1)
for i =1:size(Xr,1)-1
    B_S = B_S + (2 * delta_X_r(i,1)*delta_X_ba(i,:) + 2 * delta_Y_r(i,1) * delta_Y_ba(i,:)) *  E(2*i-1:2*i,:);
end

% objective function of minimum curvature
H_tao = dx' * (D' * D) * dx + dy' * (D' * D) * dy;
B_tao = 2*Xr'*(D'*D)*dx + 2*Yr'*(D'*D)*dy;

% objective function of centering driving
w1 = zeros(size(Xr,1)-1,size(Xr,1));
for i = 1:size(Xr,1)-1
    w1(i,i) = 1;
end

w2 = zeros(size(Xr,1)-1,size(Xr,1));
for i = 1:size(Xr,1)-1
    w2(i,i+1) = 1;
end

H_P = (w1 - w2)' * (w1 - w2);%(n+1)*(n+1)
B_P = zeros(1,size(Xr,1));

% Quadratic programming
H = H_S * 2;
f = B_S';
% lb = zeros(size(Xr,1),1);
lb = 0.2*ones(size(Xr,1),1);
ub = 0.8*ones(size(Xr,1),1);
lb(1:3) = Init_pos;
ub(1:3)=Init_pos;
lb(end-2:end) = Init_pos;
ub(end-2:end)=Init_pos;
%     lb(end) = 0.5;
%     ub(end) = 0.5;
alpha_path_length = activeset_bc_simple(H,f,lb,ub);

H = 2*H_tao;
f = B_tao';
alpha_curvature = activeset_bc_simple(H,f,lb,ub);

alpha_centering=0.5*ones(size(Xr,1),1);
alpha_centering(1) = Init_pos;
%     alpha_centering(2:end) = 0.5;

H = 2*H_P;
f = B_P';
alpha_heading_error = activeset_bc_simple(H,f,lb,ub);
%alpha_heading_error = quadprog(H,f,[],[],[],[],lb,ub,[],options);
    
%     alpha = beta_path_length*alpha1 + beta_curvature*alpha2 + beta_centering*alpha3 + (1-beta_path_length-beta_curvature-beta_centering)*alpha4;
end


function cur_fro = Curvature_cal(XtsTem,YtsTem)
coder.extrinsic('smooth');
Num_path=size(XtsTem,2);
cur_fro = zeros(size(XtsTem));
span = 6;% used to smooth the curvature
for j=1:Num_path
    for i = 1:size(XtsTem,1)
        if (i == 1)
            x = [XtsTem(i,j);XtsTem(i+1,j);XtsTem(i+2,j);XtsTem(i+3,j);XtsTem(i+4,j)];
            y = [YtsTem(i,j);YtsTem(i+1,j);YtsTem(i+2,j);YtsTem(i+3,j);YtsTem(i+4,j)];
        elseif (i == 2)
            x = [XtsTem(i-1,j);XtsTem(i,j);XtsTem(i+1,j);XtsTem(i+2,j);XtsTem(i+3,j)];
            y = [YtsTem(i-1,j);YtsTem(i,j);YtsTem(i+1,j);YtsTem(i+2,j);YtsTem(i+3,j)];
        elseif (i == size(XtsTem,1)-1)
            x = [XtsTem(i-3,j);XtsTem(i-2,j);XtsTem(i-1,j);XtsTem(i,j);XtsTem(i+1,j)];
            y = [YtsTem(i-3,j);YtsTem(i-2,j);YtsTem(i-1,j);YtsTem(i,j);YtsTem(i+1,j)];
        elseif (i == size(XtsTem,1))
            x = [XtsTem(i-4,j);XtsTem(i-3,j);XtsTem(i-2,j);XtsTem(i-1,j);XtsTem(i,j)];
            y = [YtsTem(i-4,j);YtsTem(i-3,j);YtsTem(i-2,j);YtsTem(i-1,j);YtsTem(i,j)];
        else
            x = [XtsTem(i-2,j);XtsTem(i-1,j);XtsTem(i,j);XtsTem(i+1,j);XtsTem(i+2,j)];
            y = [YtsTem(i-2,j);YtsTem(i-1,j);YtsTem(i,j);YtsTem(i+1,j);YtsTem(i+2,j)];
        end
%             cur_fro(i,j) = rwqulv(x,y); 
        A=[x,y,ones(length(x),1)];
        if rank(A) ~= size(A,2)
            cur_fro(i,j) = 0;
        else
            B=-1*(x.^2+y.^2);
            coef=A\B;%圆一般方程式的的系数DEF
            cur_fro(i,j)= 2/sqrt(coef(1)^2+coef(2)^2-4*coef(3));
        end
    end  
    cur_fro(:,j)= smooth(cur_fro(:,j),span);
end
end


function Speed_PlannedTemp=Speedprofile(Num_point,Curvature,a_latlim,a_acclim,a_declim,v_min_con,v_max_con,G)

coder.extrinsic('quadprog','optimoptions');  
% lb_1 = [];
% ub_1 = [];
miu=0.8;% the Road adhesion coefficient
g=9.8;% m/s2,the Gravity coefficient
v_max_TierAdLimit=sqrt(miu * g ./ (Curvature+eps));%upper bounds by tier adhesion limit
ub_Curvature = sqrt(1 ./ (abs(Curvature)+eps) .* a_latlim);% upper bounds by Parameter_LatAcceleration
ub_Parameter = v_max_con .* ones(Num_point,1);%speed upper bound from Parameter_SpeedPlan
lb_Parameter = v_min_con .* ones(Num_point,1);%speed lower bound from Parameter_SpeedPlan

UpperBound =min([ub_Curvature,ub_Parameter],[],2);
UpperBound=max([UpperBound,lb_Parameter],[],2)+0.1;
LowerBound = lb_Parameter;

v_MaxTarget = min(v_max_TierAdLimit,ub_Parameter);
H_QuadObjective = 2 * eye(Num_point);% quadratic obejective term
f_LinearObjective = -2 * v_MaxTarget';% Linear obejective term
A_InequallityConstraint = [G.*2;-G.*2];% Linear inequallity constraints
b_InequallityConstraint= [a_acclim .* ones(Num_point,1);a_declim .* ones(Num_point,1)];% Linear Inequality constraints
% Speed_Planned=zeros(1000,1);
options = optimoptions('quadprog','Display','off');
Speed_PlannedTemp = quadprog(H_QuadObjective,f_LinearObjective,A_InequallityConstraint,b_InequallityConstraint,[],[],LowerBound,UpperBound,[],options);% There is no equality constraints 
% Speed_Planned(1:Num_point,1)=Speed_PlannedTemp;

end

function x=activeset_bc_simple(H,g,LB,UB)
%
% Active set algorithm for quadratic program with bound constraints. 
% [x,lam,ws,oc,cc]=activeset_bc(H,g,LB,UB,tol,maxiter), solves the 
% strictly convex quadratic program of the form
%
% min 0.5x'*H*x+g'*x, s.t. LB<=x<=UB, 
%
% where H=H'>0. 
%
% [x,lam,ws,oc,cc]=activeset_bc(H,g,LB,UB), work with default parameters.
% 
% This is modification of the algorithm 16.3 from Nocedal & Wright , p. 472.
% Input:
% H - positive definite and symmetric hessian matrix (nxn).
% g - vetor (nx1).
% tol - tolerance for equality constrained subproblem (16.39), p. 468 in N&W, (Default: 10^(-12)) 
% maxiter - max. number of main iterations, (Default: 100*length(x))
% Output: 
% x  - optimal solution.
% f=0.5x'*H*x+g'*x - minimum function value 
% lam(k) - Lagrange multiplier corresponding to LB(k)<=x(k)<=UB(k), k=1,..,n.
% ws - is an optimal active set. If ws(k)=-1, then x(k)=LB(k). If ws(k)=+1,
% then x(k)=UB(k), otherwise ws(k)=0.
% oc - is an optimality measure i.e. ||Lx||=||H*x+g-A'*lam||, where
% the Lagrangian
%
% L=0.5x'*H*x+g'*x-lam'*(A*x-b),
%
% and A=[I;-I], b=[LB;-UB].
%
% cc - is complementarity measure i.e.
%
% cc = max  |lam(i)*min(x(i)-LB(i),UB(i)-x(i))|
%    i=1,..,n
%
% The activeset_bc, is usually (but not always), faster than quadprog/interior-point 
% To compare with quadprog/interior-point try to run the following code:

% (C) 2021, by dr Piotr Bania, pba@agh.edu.pl.
% http://home.agh.edu.pl/~pba/

n=length(g);
LB=LB(:);UB=UB(:);g=g(:);
[nh,mh]=size(H);nlb=length(LB);nub=length(UB);
s=(nh==mh && n==nh && n==nub && n==nlb);
if ~s
    x=0.5*ones(n,1);
    return
end
tol=1e-10;
maxiter=100*n;

k=0;stop=0;
opts.SYM =true;opts.POSDEF=true;opts.TRANSA=false;
x=linsolve(H,-g,opts); % Compute global solution.
x=max(LB,x);x=min(UB,x); % Starting point.
% Working set. 
% If x(k)=LB(k)-->ws(k)=-1, elseif x(k)=UB(k)-->ws(k)=+1,else --> ws(k)=0. 
ws=zeros(n,1);ws(x==LB)=-1;ws(x==UB)=1;
% If ws is empty -->stop, global solution LB<x=-H^(-1)g<UB.
if max(abs(ws))==0
    stop=1;
end
while ~stop
    gk=H*x+g; % Compute gradient.
    ind=find(ws==0); % Identify free variables.
    if isempty(ind) % If all constraints are active.
        % Trivial solution of the equality constrained subproblem. 
        pk=zeros(n,1);
        lam=-ws.*gk; % Compute Lagrange multipliers.
    else
        % Solution of the equality constrained subproblem.
        Hr=H(ind,ind);gr=gk(ind); % Reduced hessian and gradient. 
        pr=linsolve(Hr,-gr,opts); % Solution of the reduced subproblem. 
        pk=zeros(n,1);pk(ind)=pr; % Solution of the subproblem. 
        lam=-ws.*(H*pk+gk); % Compute Lagrange multipliers, A'*lam=H*pk+gk.
    end
    if norm(pk)<tol % If pk==0, i.e. the subproblem has trivial solution.
        if min(lam)>=0  
            stop=1; % If all multipliers are non-negative --> stop.
        else
            ws(lam<0)=0; % Remove constraints with negative multipliers.
        end
    else
        % Max step and blocking constraint
        [al,jblock,sg]=get_max_step(x,pk,LB,UB,n);
        if jblock>0 % If there are some blocking constraint.
            ws(jblock)=sg; % Add blocking constraint to ws.
        end
        x=x+al*pk; % Step
    end
    k=k+1;
    if k>maxiter % If max. number of iteration
        stop=1;
    end
end
end
%% 
function [al,j,s]=get_max_step(x,pk,LB,UB,n)
% Compute max. step s.t LB<=x+al*pk<=UB && 0<=al<=1.
% j - index of blocking constraint,
% s=1, upper bound is active , s=-1 - lower bound is active
% If LB<x+pk<UB, then al=1, j=0, s=0 - no blocking constraits
al=1;j=0;s=0;
for i=1:n
    if pk(i)>0
        altmp=(UB(i)-x(i))/pk(i);stmp=1;
    elseif pk(i)<0
        altmp=(LB(i)-x(i))/pk(i);stmp=-1;
    else
        altmp=inf;stmp=0;
    end
    if altmp<al
        al=altmp;j=i;s=stmp;  
    end
end
end
